simulink model "planttest"  (R2024b)
settings: Solver=VariableStepAuto  StartTime=0.0  StopTime=10.0  RelTol=1e-3
values from neighbouring files (symbols this model uses):
  Dm2 = 0    [SimParameters.m]    (also in param.mat)
  Dm3 = 0    [SimParameters.m]    (also in param.mat)
  Jm2 = 4.6370e-04    (= 0.0004637)    [SimParameters.m]    (also in param.mat)
  Jm3 = 2.4640e-04    (= 0.0002464)    [SimParameters.m]    (also in param.mat)
  Kpp2 = 2.0    (= 2)    [SimParameters.m]    (also in param.mat = 10)
  Kpp3 = 2.0    (= 2)    [SimParameters.m]    (also in param.mat = 10)
  Kt2 = (0.07354) * (4)    (= 0.29416)    [SimParameters.m]    (also in param.mat)
  Kt3 = (0.0631765) * (4)    (= 0.252706)    [SimParameters.m]    (also in param.mat)
  Kvi2 = (w2*w2*Jm2)/Kt2    (= 3.94088251292)    [SimParameters.m]    (also in param.mat)
  Kvi3 = (w3*w3*Jm3)/Kt3    (= 2.43761525251)    [SimParameters.m]    (also in param.mat)
  Kvp2 = (Jm2*w2*zeta2)/Kt2    (= 0.0788176502584)    [SimParameters.m]    (also in param.mat)
  Kvp3 = (Jm3*w3*zeta3)/Kt3    (= 0.0487523050501)    [SimParameters.m]    (also in param.mat)
settings Model: Creator=TatsudaKenta  LastModifiedBy=TatsudaKenta

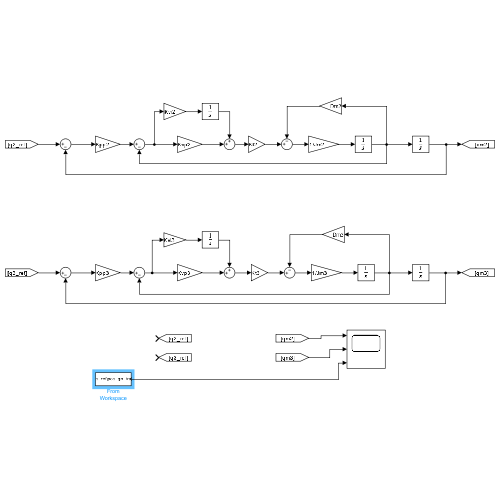
[thumbnail: Simulink's stored preview of the top-level diagram]
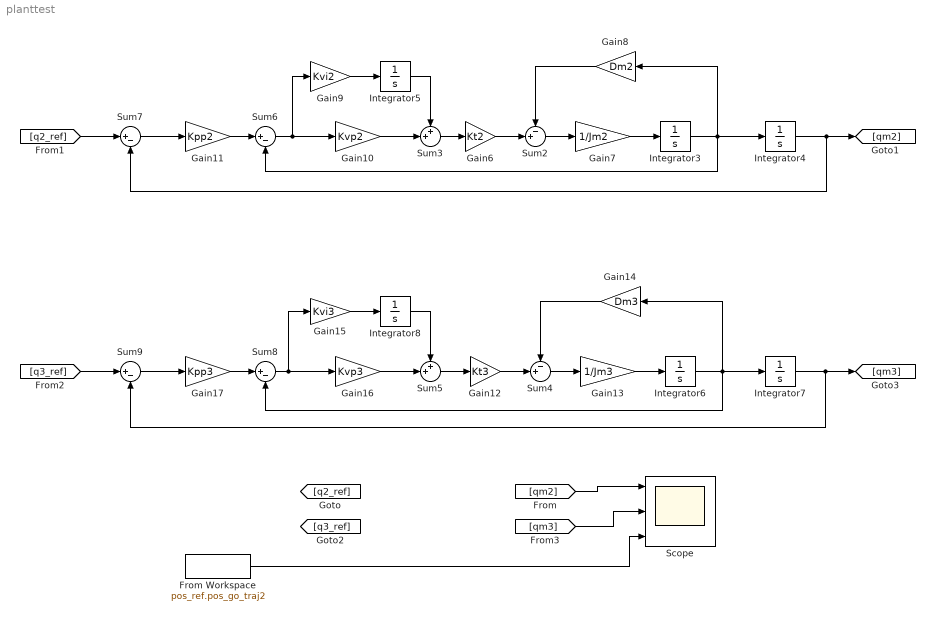
== system planttest ==
  From Workspace : FromWorkspace  VariableName=pos_ref.pos_go_traj2
  Gain10 : Gain  Gain=Kvp2
  Gain11 : Gain  Gain=Kpp2
  Gain12 : Gain  Gain=Kt3
  Gain13 : Gain  Gain=1/Jm3
  Gain14 : Gain  Gain=Dm3
  Gain15 : Gain  Gain=Kvi3
  Gain16 : Gain  Gain=Kvp3
  Gain17 : Gain  Gain=Kpp3
  Gain6 : Gain  Gain=Kt2
  Gain7 : Gain  Gain=1/Jm2
  Gain8 : Gain  Gain=Dm2
  Gain9 : Gain  Gain=Kvi2
  Integrator{3..8} (6 alike) : Integrator
  Scope : Scope  NumInputPorts=3
  Sum2 : Sum  Inputs=-+|
  Sum3 : Sum  Inputs=++|
  Sum4 : Sum  Inputs=-+|
  Sum5 : Sum  Inputs=++|
  Sum{6..9} (4 alike) : Sum  Inputs=|+-
  wires:
  [qm2] -> Scope/1
  [qm3] -> Scope/2
  Gain11/1 -> Sum6/1
  Integrator7/1 -> [qm3], Sum9/2
  Gain17/1 -> Sum8/1
  Sum5/1 -> Gain12/1
  Gain13/1 -> Integrator6/1
  Integrator8/1 -> Sum5/1
  Sum6/1 -> Gain9/1, Gain10/1
  Sum8/1 -> Gain15/1, Gain16/1
  Gain10/1 -> Sum3/2
  Gain15/1 -> Integrator8/1
  Gain16/1 -> Sum5/2
  [q2_ref] -> Sum7/1
  Gain12/1 -> Sum4/2
  Sum4/1 -> Gain13/1
  Integrator5/1 -> Sum3/1
  Sum9/1 -> Gain17/1
  Gain14/1 -> Sum4/1
  Integrator4/1 -> Sum7/2, [qm2]
  [q3_ref] -> Sum9/1
  Integrator6/1 -> Sum8/2, Gain14/1, Integrator7/1
  Gain9/1 -> Integrator5/1
  Sum7/1 -> Gain11/1
  Sum3/1 -> Gain6/1
  Gain7/1 -> Integrator3/1
  Integrator3/1 -> Sum6/2, Integrator4/1, Gain8/1
  Sum2/1 -> Gain7/1
  Gain6/1 -> Sum2/2
  Gain8/1 -> Sum2/1
  From Workspace/1 -> Scope/3
